simulink model "LMI_lema_8_statefeedback_robusto"  (Simulink 7.7)
settings: Solver=ode45  StartTime=0.0  StopTime=50  RelTol=1e-3
values from neighbouring files (symbols this model uses):
  QT =     [FaseMinima.mat]    (also in FaseNaoMinima.mat; FaseNaoMinimaMudandoApenasGama.mat; settup.m = dynamics())
settings Model: Creator=Arthur  LastModifiedBy=Arthur
settings DebuggingCC: UnderspecifiedInitializationDetection=Simplified

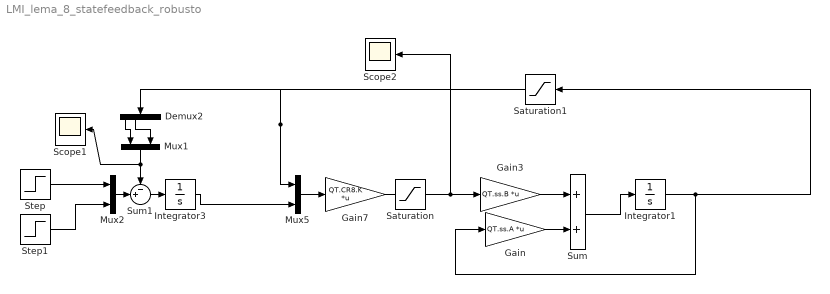
== system LMI_lema_8_statefeedback_robusto ==
  Demux2 : Demux
  Gain : Gain  Gain=QT.ss.A  Multiplication=Matrix(K*u)
  Gain3 : Gain  Gain=QT.ss.B  Multiplication=Matrix(K*u)
  Gain7 : Gain  Gain=QT.CR8.K  Multiplication=Matrix(K*u)
  Integrator1 : Integrator
  Integrator3 : Integrator
  Mux1 : Mux  Inputs=2
  Mux2 : Mux  Inputs=2
  Mux5 : Mux  Inputs=2
  Saturation : Saturate  UpperLimit=1.5  LowerLimit=-1.5
  Saturation1 : Saturate  UpperLimit=20  LowerLimit=0
  Scope1 : Scope
      settings: TimeRange=100  YMin=0  YMax=1  SampleTime=1
  Scope2 : Scope
      settings: TimeRange=100  YMin=0  YMax=1  SampleTime=1
  Step : Step  SampleTime=0
  Step1 : Step  Time=10  After=2  SampleTime=0
  Sum : Sum
  Sum1 : Sum  Inputs=-+|
  wires:
  Gain/1 -> Sum/2
  Gain3/1 -> Sum/1
  Step/1 -> Mux2/1
  Step1/1 -> Mux2/2
  Integrator1/1 -> Gain/1, Saturation1/1
  Sum/1 -> Integrator1/1
  Gain7/1 -> Gain3/1, Scope2/1
  Mux5/1 -> Gain7/1
  Integrator3/1 -> Mux5/2
  Sum1/1 -> Integrator3/1
  Mux2/1 -> Sum1/2
  Demux2/1 -> Mux1/1
  Demux2/2 -> Mux1/2
  Mux1/1 -> Sum1/1, Scope1/1
  Saturation1/1 -> Mux5/1, Demux2/1
